simulink model "xCarre"  (R2016b)
settings: Solver=VariableStepAuto  StartTime=0  StopTime=2  RelTol=1e-3
settings Model: Creator=live  LastModifiedBy=live

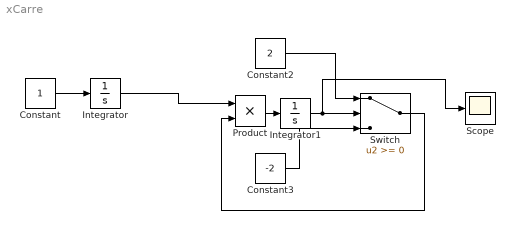
== system xCarre ==
  Constant : Constant
  Constant2 : Constant  Value=2
  Constant3 : Constant  Value=-2
  Integrator : Integrator  InitialCondition=-1
  Integrator1 : Integrator  InitialCondition=1
  Product : Product
  Scope : Scope
  Switch : Switch
  wires:
  Constant/1 -> Integrator/1
  Integrator/1 -> Product/1
  Constant2/1 -> Switch/1
  Constant3/1 -> Switch/3
  Product/1 -> Integrator1/1
  Integrator1/1 -> Scope/1, Switch/2
  Switch/1 -> Product/2
